simulink model "rc_krets"  (R2017a)
settings: Solver=VariableStepAuto  StartTime=0.0  StopTime=10.0  RelTol=1e-3
values from neighbouring files (symbols this model uses):
  C = 100*10^-6    (= 0.0001)    [par11.m]
  R = 10000    [par11.m]
settings Model: Creator=bruker  LastModifiedBy=bruker

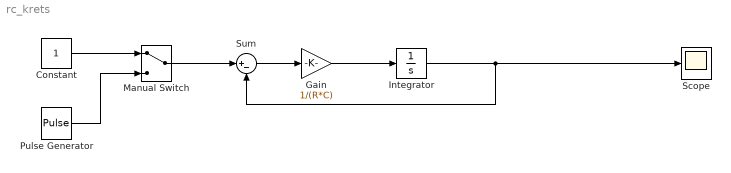
== system rc_krets ==
  Constant : Constant
  Gain : Gain  Gain=1/(R*C)
  Integrator : Integrator
  Manual Switch : ManualSwitch
  Pulse Generator : DiscretePulseGenerator  PulseType=Time based  Amplitude=100  Period=10  PulseWidth=0.1  PhaseDelay=2
  Scope : Scope
  Sum : Sum  Inputs=|+-
  wires:
  Sum/1 -> Gain/1
  Gain/1 -> Integrator/1
  Integrator/1 -> Sum/2, Scope/1
  Manual Switch/1 -> Sum/1
  Constant/1 -> Manual Switch/1
  Pulse Generator/1 -> Manual Switch/2
